simulink model "L4_simulnk"  (R2023b)
settings: Solver=VariableStepAuto  StartTime=0.0  StopTime=5  RelTol=1e-3
settings Model: Creator=Salvador  LastModifiedBy=Salvador

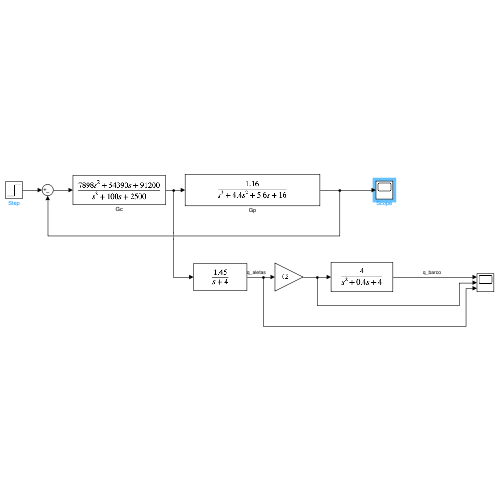
[thumbnail: Simulink's stored preview of the top-level diagram]
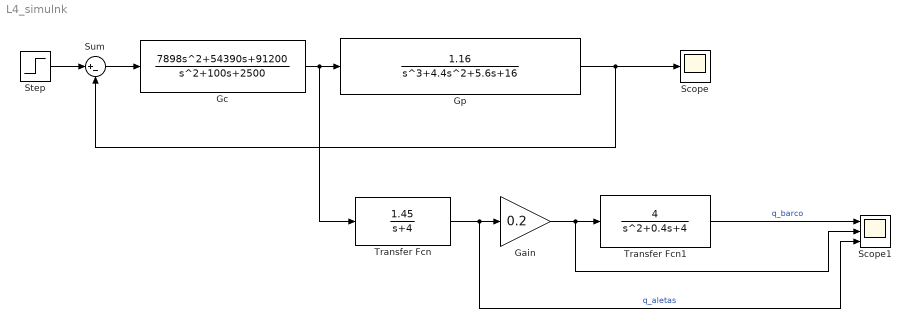
== system L4_simulnk ==
  Gain : Gain  Gain=0.2
  Gc : TransferFcn  Numerator=[7898 54390 91200]  Denominator=[1 100 2500]
  Gp : TransferFcn  Numerator=[1.16]  Denominator=[1 4.4 5.6 16]
  Scope : Scope
  Scope1 : Scope  NumInputPorts=3
  Step : Step  Time=0  After=0.1  SampleTime=0
  Sum : Sum  Inputs=|+-
  Transfer Fcn : TransferFcn  Numerator=[1.45]  Denominator=[1 4]
  Transfer Fcn1 : TransferFcn  Numerator=[4]  Denominator=[1 0.4 4]
  wires:
  Gc/1 -> Transfer Fcn/1, Gp/1
  Gp/1 -> Scope/1, Sum/2
  Sum/1 -> Gc/1
  Step/1 -> Sum/1
  Transfer Fcn/1 -> Scope1/3, Gain/1  "q_aletas"
  Gain/1 -> Scope1/2, Transfer Fcn1/1
  Transfer Fcn1/1 -> Scope1/1  "q_barco"
